simulink model "TrabalhoRedesSimulink"  (R2012b)
settings: Solver=ode45  StartTime=0.0  StopTime=10.0  RelTol=1e-3
libraries: commrandsrc2 x1, commfilt2 x1
settings Model: Creator=André  LastModifiedBy=André

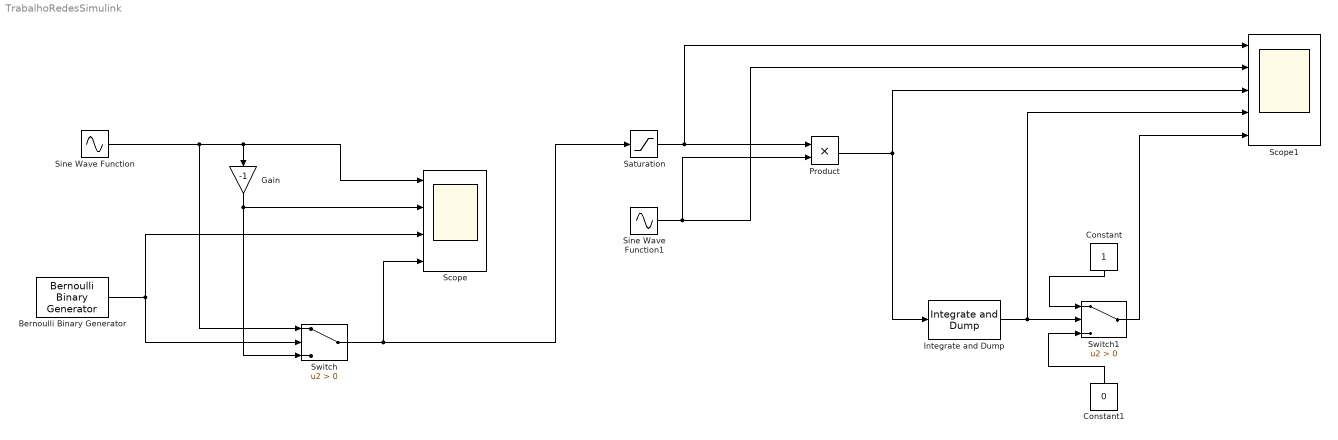
== system TrabalhoRedesSimulink ==
  Bernoulli Binary Generator : commrandsrc2/Bernoulli Binary Generator  P=0.5  seed=14  Ts=1  frameBased=off  sampPerFrame=1  orient=off  outDataType=double
  Constant : Constant
  Constant1 : Constant  Value=0
  Gain : Gain  Gain=-1
  Integrate and Dump : commfilt2/Integrate and Dump  obssamples=8  offsetsamples=0  nodump=off  roundingMode=Floor  overflowMode=off
  Product : Product  RndMeth=Zero
  Saturation : Saturate
  Scope : Scope  NumInputPorts=4
      settings: YMin=-5~-5~-5~-5  YMax=5~5~5~5
  Scope1 : Scope  NumInputPorts=5
      settings: YMin=-5~-5~-5~-5~-5  YMax=5~5~5~5~5
  Sine Wave Function : Sin  SineType=Sample based  Amplitude=2  Frequency=1000  Samples=100  SampleTime=0.01
  Sine Wave Function1 : Sin  SineType=Sample based  Amplitude=2  Frequency=1000  Samples=100  SampleTime=0.01
  Switch : Switch  Criteria=u2 > Threshold
  Switch1 : Switch  Criteria=u2 > Threshold
  wires:
  Sine Wave Function/1 -> Switch/1, Scope/1, Gain/1
  Gain/1 -> Switch/3, Scope/2
  Bernoulli Binary Generator/1 -> Scope/3, Switch/2
  Switch/1 -> Scope/4, Saturation/1
  Saturation/1 -> Scope1/1, Product/1
  Sine Wave Function1/1 -> Product/2, Scope1/2
  Product/1 -> Integrate and Dump/1, Scope1/3
  Constant/1 -> Switch1/1
  Constant1/1 -> Switch1/3
  Integrate and Dump/1 -> Scope1/4, Switch1/2
  Switch1/1 -> Scope1/5
